simulink model "dev_lab7"  (Simulink 8.6)
settings: Solver=ode3  StartTime=0  StopTime=2.5  FixedStep=Ts  RelTol=1e-5
values from neighbouring files (symbols this model uses):
  Ac = 5    [dev_digicomm_lab7.m]    (also in qam4-plotted.m)
  fs = 1/Ts    (= 2000000)    [dev_digicomm_lab7.m]    (also in qam4-plotted.m)
  rc = fc*2*pi    (= 125663.706144)    [dev_digicomm_lab7.m]    (also in qam4-plotted.m)
  Tb = 250E-6    (= 0.00025)    [dev_digicomm_lab7.m]    (also in qam4-plotted.m)
  Ts = Tb/500    (= 5e-07)    [dev_digicomm_lab7.m]    (also in qam4-plotted.m)
libraries: commfilt2 x2, commchan3 x1, commsink2 x1, commrandsrc2 x1
settings Model: Creator=Dennis Silage  LastModifiedBy=trejo  SimulationMode=accelerator
settings OptimizationCC: InitFltsAndDblsToZero=on
settings DebuggingCC: SolverPrmCheckMsg=none  FcnCallInpInsideContextMsg=UseLocalSettings
settings GRTTargetCC: GeneratePreprocessorConditionals=Use local settings

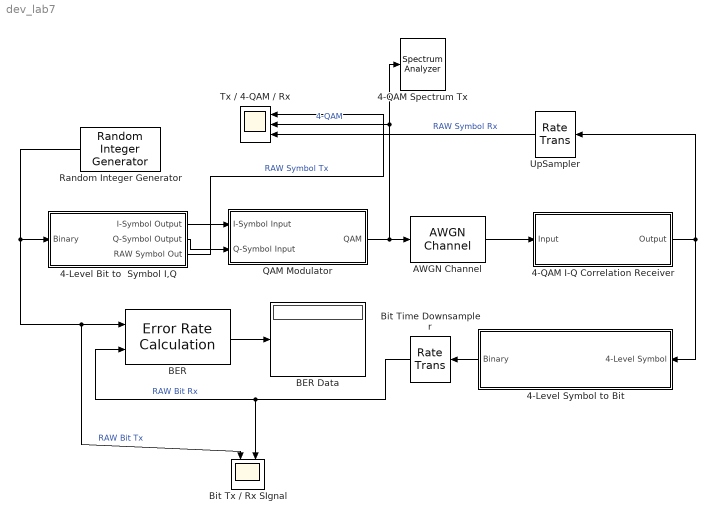
== system dev_lab7 ==
  4-Level Bit to  Symbol I,Q : Subsystem
  4-Level Symbol to Bit : Subsystem
  4-QAM Spectrum Tx : SpectrumAnalyzer
  4-QAM I-Q Correlation Receiver : Subsystem
  AWGN Channel : commchan3/AWGN Channel  InputProcessing=Inherited (this choice will be removed - see release notes)  seed=randseed  noiseMode=Variance from mask  EbNodB=12  EsNodB=12  SNRdB=SNR  bitsPerSym=2  Ps=50  Tsym=Tb*2  variance=N0
  BER : commsink2/Error Rate Calculation  N=6  st_delay=0  cp_mode=Entire frame  subframe=[]  PMode=Port  WsName=ErrorVec  RsMode2=off  stop=off  numErr=100  maxBits=1e6
  BER Data : Display
  "Bit Time Downsampler  " : RateTransition  OutPortSampleTime=Tb
  Bit Tx / Rx SIgnal : Scope  NumInputPorts=2
  QAM Modulator : Subsystem
  Random Integer Generator : commrandsrc2/Random Integer Generator  mul=2  seed=randseed  Ts=Tb  frameBased=off  sampPerFrame=1  orient=off  outDataType=double
  Tx / 4-QAM / Rx : Scope  NumInputPorts=3
  UpSampler : RateTransition  OutPortSampleTime=Ts
  wires:
  BER/1 -> BER Data/1
  4-Level Symbol to Bit/1(Binary) -> "Bit Time Downsampler  "/1
  4-QAM I-Q Correlation Receiver/1(Output) -> UpSampler/1, 4-Level Symbol to Bit/1(4-Level Symbol)
  4-Level Bit to  Symbol I,Q/1(I-Symbol Output) -> QAM Modulator/1(I-Symbol Input)
  4-Level Bit to  Symbol I,Q/2(Q-Symbol Output) -> QAM Modulator/2(Q-Symbol Input)
  QAM Modulator/1(QAM) -> AWGN Channel/1, 4-QAM Spectrum Tx/1, Tx / 4-QAM / Rx/2  "4-QAM"
  UpSampler/1 -> Tx / 4-QAM / Rx/3  "RAW Symbol Rx"
  4-Level Bit to  Symbol I,Q/3("RAW Symbol Out ") -> Tx / 4-QAM / Rx/1  "RAW Symbol Tx"
  "Bit Time Downsampler  "/1 -> Bit Tx / Rx SIgnal/2, BER/2  "RAW Bit Rx"
  Random Integer Generator/1 -> 4-Level Bit to  Symbol I,Q/1(Binary), Bit Tx / Rx SIgnal/1, BER/1  "RAW Bit Tx"
  AWGN Channel/1 -> 4-QAM I-Q Correlation Receiver/1(Input)

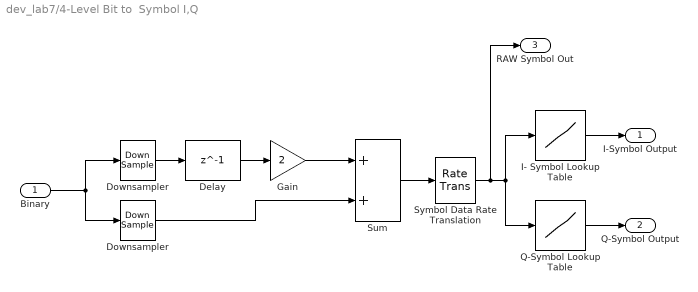
== system dev_lab7/4-Level Bit to  Symbol I,Q ==
  Binary : Inport
  Delay : Delay  DelayLength=1  InitialCondition=0  InputProcessing=Inherited
  Downsampler : DownSample  InputProcessing=Inherited (this choice will be removed - see release notes)  smode=Force single rate  fmode=Maintain input frame rate
  "Downsampler " : DownSample  phase=1  InputProcessing=Inherited (this choice will be removed - see release notes)  smode=Force single rate  fmode=Maintain input frame rate
  Gain : Gain  Gain=2
  I- Symbol Lookup Table : Lookup  InputValues=[0,1,2,3]  Table=[0,1,-1,0]  LookUpMeth=Use Input Nearest
  Q-Symbol Lookup Table : Lookup  InputValues=[0,1,2,3]  Table=[0,3,3,-3]  LookUpMeth=Use Input Nearest
  Sum : Sum
  Symbol Data Rate Translation : RateTransition  OutPortSampleTime=Ts
  I-Symbol Output : Outport
  Q-Symbol Output : Outport  Port=2
  "RAW Symbol Out " : Outport  Port=3
  wires:
  Delay/1 -> Gain/1
  Downsampler/1 -> Delay/1
  Binary/1 -> "Downsampler "/1, Downsampler/1
  Gain/1 -> Sum/1
  "Downsampler "/1 -> Sum/2
  Sum/1 -> Symbol Data Rate Translation/1
  Q-Symbol Lookup Table/1 -> Q-Symbol Output/1
  I- Symbol Lookup Table/1 -> I-Symbol Output/1
  Symbol Data Rate Translation/1 -> "RAW Symbol Out "/1, I- Symbol Lookup Table/1, Q-Symbol Lookup Table/1

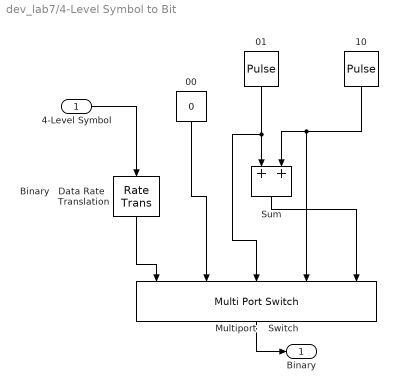
== system dev_lab7/4-Level Symbol to Bit ==
  4-Level Symbol : Inport
  "   Multiport    Switch" : MultiPortSwitch  DataPortOrder=Zero-based contiguous  Inputs=4  zeroidx=on
  "00 " : Constant  Value=0
  "01 " : DiscretePulseGenerator  Period=2*Tb*fs  PulseWidth=Tb*fs  PhaseDelay=Tb*fs  SampleTime=Ts  VectorParams1D=off
  "10 " : DiscretePulseGenerator  Period=2*Tb*fs  PulseWidth=Tb*fs  SampleTime=Ts
  "Binary   Data Rate   Translation  " : RateTransition  OutPortSampleTime=Ts
  Sum : Sum
  Binary : Outport
  wires:
  "   Multiport    Switch"/1 -> Binary/1
  "00 "/1 -> "   Multiport    Switch"/2
  "01 "/1 -> "   Multiport    Switch"/3, Sum/1
  Sum/1 -> "   Multiport    Switch"/5
  4-Level Symbol/1 -> "Binary   Data Rate   Translation  "/1
  "Binary   Data Rate   Translation  "/1 -> "   Multiport    Switch"/1
  "10 "/1 -> Sum/2, "   Multiport    Switch"/4

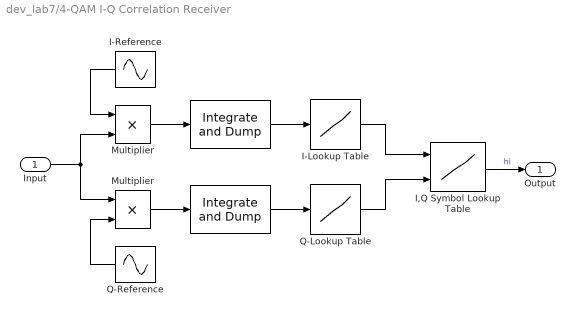
== system dev_lab7/4-QAM I-Q Correlation Receiver ==
  Input : Inport
  " " : commfilt2/Integrate and Dump  obssamples=2*Tb*fs  offsetsamples=0  nodump=off  roundingMode=Floor  overflowMode=off
  "  " : commfilt2/Integrate and Dump  obssamples=2*Tb*fs  offsetsamples=0  nodump=off  roundingMode=Floor  overflowMode=off
  I,Q Symbol Lookup Table : Lookup2D  RowIndex=[1,2,3]  ColumnIndex=[1,2,3]  Table=[0 0 2; 3 0 0; 0 0 1]  LookUpMeth=Use Input Nearest
  I-Lookup Table : Lookup  InputValues=[-3000,0,3000]  Table=[1,2,3]  LookUpMeth=Use Input Nearest
  I-Reference : Sin  Amplitude=Ac  Frequency=rc  Phase=pi/2  SampleTime=Ts
  Multiplier : Product  RndMeth=Zero
  "Multiplier " : Product  RndMeth=Zero
  Q-Lookup Table : Lookup  InputValues=[-3000,0,3000]  Table=[1,2,3]  LookUpMeth=Use Input Nearest
  Q-Reference : Sin  Amplitude=Ac  Frequency=rc  SampleTime=Ts
  Output : Outport
  wires:
  I-Lookup Table/1 -> I,Q Symbol Lookup Table/1
  Q-Lookup Table/1 -> I,Q Symbol Lookup Table/2
  I,Q Symbol Lookup Table/1 -> Output/1  "hi"
  I-Reference/1 -> "Multiplier "/1
  Q-Reference/1 -> Multiplier/2
  Input/1 -> "Multiplier "/2, Multiplier/1
  Multiplier/1 -> "  "/1
  "  "/1 -> Q-Lookup Table/1
  "Multiplier "/1 -> " "/1
  " "/1 -> I-Lookup Table/1

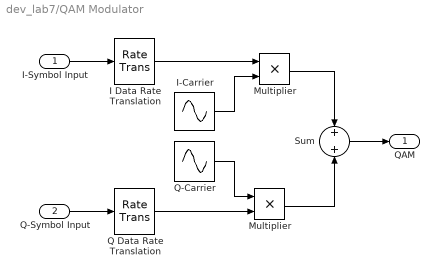
== system dev_lab7/QAM Modulator ==
  I-Symbol Input : Inport
  Q-Symbol Input : Inport  Port=2
  " Multiplier " : Product  RndMeth=Zero
  I Data Rate Translation : RateTransition  OutPortSampleTime=Ts
  I-Carrier : Sin  Amplitude=Ac  Frequency=rc  Phase=pi/2  SampleTime=Ts  VectorParams1D=off
  Multiplier : Product  RndMeth=Zero
  Q Data Rate Translation : RateTransition  OutPortSampleTime=Ts
  Q-Carrier : Sin  Amplitude=Ac  Frequency=rc  SampleTime=Ts  VectorParams1D=off
  Sum : Sum
  QAM : Outport
  wires:
  I Data Rate Translation/1 -> Multiplier/1
  Q Data Rate Translation/1 -> " Multiplier "/2
  I-Carrier/1 -> Multiplier/2
  Q-Carrier/1 -> " Multiplier "/1
  Multiplier/1 -> Sum/1
  " Multiplier "/1 -> Sum/2
  Sum/1 -> QAM/1
  I-Symbol Input/1 -> I Data Rate Translation/1
  Q-Symbol Input/1 -> Q Data Rate Translation/1
